simulink model "Motor_Cmd_varY_eqHarness"  (Simulink 7.9)
settings: Solver=FixedStepDiscrete  StartTime=0.0  StopTime=10  RelTol=1e-3
PreLoadFcn:
  | Motor_Cmd_varY_selfinit
undefined symbols (not defined in the file): sigbuilder_block
libraries: simulink x1
settings Model: RequirementInfo="{}  %GIDa_76f203d0_57c5_4172_aee2_9207869380ab"  SldvGeneratedHarnessModel=TestUnitModel=Motor_Cmd_varY|  Creator=fguerin  LastModifiedBy=klindqvi  CovMetricSettings=dcmoe  CovHTMLOptions=-aTS=1 -bRG=1 -bTC=0 -hTR=0 -nFC=0 -scm=1 -bcm=1  CovModelRefEnable=on  CovExternalEMLEnable=on
settings DataIOCC: ExternalInput=[t,u]  LimitDataPoints=off  SaveFormat=StructureWithTime  SaveOutput=off  DSMLogging=off  SaveTime=off  SignalLoggingName=logsOut
settings OptimizationCC: InlineParams=on  InlineInvariantSignals=on  EnhancedBackFolding=on  ZeroExternalMemoryAtStartup=off  ZeroInternalMemoryAtStartup=off  EfficientFloat2IntCast=on  OptimizeModelRefInitCode=on  LifeSpan=1
settings DebuggingCC: ReadBeforeWriteMsg=EnableAllAsError  WriteAfterWriteMsg=EnableAllAsError  WriteAfterReadMsg=EnableAllAsError  AlgebraicLoopMsg=error  ArtificialAlgebraicLoopMsg=error  SaveWithDisabledLinksMsg=error  SaveWithParameterizedLinksMsg=error  CheckExecutionContextPreStartOutputMsg=on  CheckExecutionContextRuntimeOutputMsg=on  BlockPriorityViolationMsg=error  SolverPrmCheckMsg=none  InheritedTsInSrcMsg=none  MultiTaskCondExecSysMsg=warning  MultiTaskRateTransMsg=warning  IntegerOverflowMsg=none  ParameterUnderflowMsg=error  ParameterPrecisionLossMsg=error  ParameterTunabilityLossMsg=error  UnderSpecifiedDataTypeMsg=warning  UnnecessaryDatatypeConvMsg=warning  VectorMatrixConversionMsg=error  SignalLabelMismatchMsg=warning  SFcnCompatibilityMsg=error  BusObjectLabelMismatch=error  RootOutportRequireBusObject=error  AssertControl=DisableAll  ModelReferenceIOMsg=error  ModelReferenceIOMismatchMessage=error  ModelReferenceCSMismatchMessage=warning  UnknownTsInhSupMsg=error  ModelReferenceDataLoggingMessage=error  ModelReferenceSymbolNameMessage=none  StrictBusMsg=ErrorOnBusTreatedAsVector
settings HardwareCC: ProdLargestAtomicInteger=Long  ProdLargestAtomicFloat=Double  ProdIntDivRoundTo=Zero  ProdEndianess=BigEndian  ProdHWDeviceType=Freescale->MPC5500
settings SFSimCC: SimParseCustomCode=off
settings RTWCC: SystemTargetFile=ert.tlc  TemplateMakefile=ert_default_tmf  Description=Embedded Coder  GenerateReport=on  RTWVerbose=off  ProcessScript=ert_make_rtw_hook  IncludeHyperlinkInReport=on  GenerateTraceInfo=on  GenerateTraceReport=on  GenerateTraceReportSl=on  GenerateTraceReportSf=on  GenerateTraceReportEml=on  GenerateCodeMetricsReport=on
settings MATStruct: className=rtw.pil.Bullseye  argsAllComponents=[]  excludedModels=[]  includeReferencedModels=on  includeTopModel=on  enabled=off
settings CodeAppCC: ForceParamTrailComments=on  IgnoreCustomStorageClasses=off  IgnoreTestpoints=on  MangleLength=4  InlinedPrmAccess=Macros  ReqsInCode=on
settings ERTTargetCC: CodeReplacementLibrary=ANSI_C  MultiwordLength=2048  SupportAbsoluteTime=off  SupportNonFinite=off  SupportComplex=off  PortableWordSizes=on  InlinedParameterPlacement=NonHierarchical  ERTCustomFileTemplate=example_file_process.tlc  ConvertIfToSwitch=off  SuppressUnreachableDefaultCases=off
settings ConfigComp: Description=Design Verifier Custom Configuration Component  DVMaxProcessTime=600  DVDisplayUnsatisfiableObjectives=on  DVAutomaticStubbing=off  DVOutputDir=C:\work\Presentations\ISO26262_workshop\newsandbox\iso26262package\WorkProducts\CodeTest  DVMakeOutputFilesUnique=off  DVTestSuiteOptimization=CombinedObjectives  DVIgnoreCovSatisfied=on  DVCoverageDataFile=C:\work\Presentations\ISO26262_workshop\newsandbox\iso26262package\WorkProducts\ModelTest\Motor_Cmd_varY_cvdata.cvt  DVDataFileName=Motor_Cmd_varY_sldvdata.mat  DVHarnessModelFileName=C:\work\Presentations\ISO26262_workshop\newsandbox\iso26262package\WorkProducts\CodeTest\Motor_Cmd_varY_eqHarness_cov  DVModelReferenceHarness=on  DVSaveReport=on  DVReportFileName=Motor_Cmd_varY_SLDV.html  DVDisplayReport=off

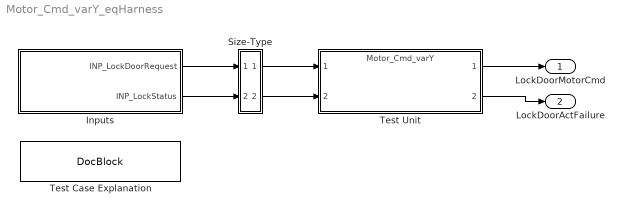
== system Motor_Cmd_varY_eqHarness ==
  Inputs : Subsystem  Tag=STV Subsys  LoadFcn=sigbuilder_block('load',[49.5 50.25 519.75 399.75 ]);  StartFcn=sigbuilder_block('start');  StopFcn=sigbuilder_block('stop');  ClipboardFcn=sigbuilder_block('clipboard');  mask(Sigbuilder block){}
      mask init:
      | if ~strcmp(get_param(bdroot(gcb),'SimulationStatus'),'stopped'),tuvar = sigbuilder_block('maskInit'); end
      settings: CopyFcn=sigbuilder_block('copy');  DeleteFcn=sigbuilder_block('delete');  ModelCloseFcn=sigbuilder_block('modelClose');  PreSaveFcn=sigbuilder_block('preSave');  NameChangeFcn=sigbuilder_block('namechange');  OpenFcn=sigbuilder_block('open');  CloseFcn=sigbuilder_block('close');
      mask Display: plot(0, 0, 100, 100,[2, 2, 32, 32, 2], [68, 8, 8, 68, 68],[32, 2], [38, 38], [32, 19, 2],[53, 60, 44], [32, 17, 17, 2],[16, 16, 31, 31]);txt = getActiveGroup(gcbh);text(2, 100, txt,'verticalAlignment', 'top');
  Size-Type : Subsystem
  Test Case Explanation : simulink/Model-Wide Utilities/DocBlock  DocumentType=Text
  Test Unit : ModelReference  ModelNameDialog=Motor_Cmd_varY  SimulationMode=Normal  ModelReferenceVersion=1.79  CopyOfModelName=Motor_Cmd_varY  DefaultDataLogging=off
  LockDoorMotorCmd : Outport  OutDataTypeStr=uint8  PortDimensions=1
  LockDoorActFailure : Outport  Port=2  OutDataTypeStr=boolean
  wires:
  Inputs/1(INP_LockDoorRequest) -> Size-Type/1(In1)
  Size-Type/1(Out1) -> Test Unit/1
  Inputs/2(INP_LockStatus) -> Size-Type/2(In2)
  Size-Type/2(Out2) -> Test Unit/2
  Test Unit/1 -> LockDoorMotorCmd/1
  Test Unit/2 -> LockDoorActFailure/1

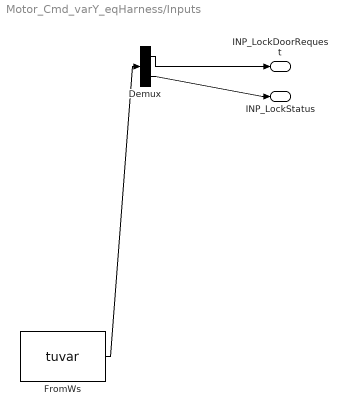
== system Motor_Cmd_varY_eqHarness/Inputs ==
  Demux : Demux  Tag=STV Demux  Outputs=2
  FromWs : FromWorkspace  Tag=STV FromWs  VariableName=tuvar  SampleTime=0  SigBuilderData=DataTag0  VnvData=DataTag1
      SigBuilderData=|
      | dataSet(1).timeRange = [0 10]
      | dataSet(1).name = 'Test1'
      | dataSet(2).timeRange = [0 10]
      | dataSet(2).name = 'Test2'
      | sbobj.Name = 'Signal Builder'
      | sbobj.Groups(1).Name = 'Test1'
      | sbobj.Groups(1).Signals(1).Name = 'INP_LockDoorRequest'
      | sbobj.Groups(1).Signals(1).XData = [0 10]
      | sbobj.Groups(1).Signals(1).YData = [0 0]
      | sbobj.Groups(1).Signals(2).Name = 'INP_LockStatus'
      | sbobj.Groups(1).Signals(2).XData = [0 10]
      | sbobj.Groups(1).Signals(2).YData = [0 0]
      | sbobj.Groups(2).Name = 'Test2'
      | sbobj.Groups(2).Signals(1).Name = 'INP_LockDoorRequest'
      | sbobj.Groups(2).Signals(1).XData = [0 1 1 2 2 10]
      | sbobj.Groups(2).Signals(1).YData = [0 0 1 1 1 1]
      | sbobj.Groups(2).Signals(2).Name = 'INP_LockStatus'
      | sbobj.Groups(2).Signals(2).XData = [0 1 1 2 2 10]
      | sbobj.Groups(2).Signals(2).YData = [0 0 0 0 1 1]
  INP_LockDoorRequest : Outport
  INP_LockStatus : Outport  Tag=STV Outport  Port=2
  wires:
  FromWs/1 -> Demux/1
  Demux/1 -> INP_LockDoorRequest/1
  Demux/2 -> INP_LockStatus/1

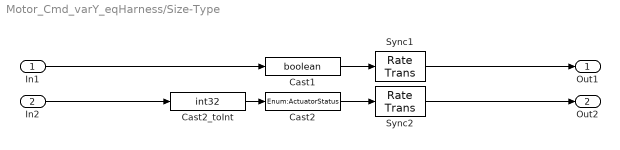
== system Motor_Cmd_varY_eqHarness/Size-Type ==
  In1 : Inport
  In2 : Inport  Port=2
  Cast1 : DataTypeConversion  OutDataTypeStr=boolean  SaturateOnIntegerOverflow=on  RndMeth=Zero
  Cast2 : DataTypeConversion  OutDataTypeStr=Enum:ActuatorStatus  SaturateOnIntegerOverflow=on  RndMeth=Zero
  Cast2_toInt : DataTypeConversion  OutDataTypeStr=int32  SaturateOnIntegerOverflow=on  RndMeth=Zero
  Sync1 : RateTransition  OutPortSampleTime=[0.20000000000000001,0]
  Sync2 : RateTransition  OutPortSampleTime=[0.20000000000000001,0]
  Out1 : Outport
  Out2 : Outport  Port=2
  wires:
  In1/1 -> Cast1/1
  Cast1/1 -> Sync1/1
  Sync1/1 -> Out1/1
  In2/1 -> Cast2_toInt/1
  Cast2_toInt/1 -> Cast2/1
  Cast2/1 -> Sync2/1
  Sync2/1 -> Out2/1
